simulink model "quadrotor_project_2021a"  (R2021a)
settings: Solver=VariableStepAuto  StartTime=0.0  StopTime=119.35  RelTol=1e-3
InitFcn:
  | sample_interval = 0.05;
  | Kp_z = 1000;
  | Kd_z = 10;
  | Kp_vel = 0.70;
  | Kd_vel = 0.2;
  | k1 = 65;
  | k2 = 25;
  | k3 = 65;
  | k4 = 25;
  | k5 = 60;
  | k6 = 55;
  | z_des = 5;
  | 
  | mdl_quadrotor;
  | J_x = quadrotor.J(1,1);
  | J_y = quadrotor.J(2,2);
  | J_z = quadrotor.J(3,3);
  | a1 = (J_y-J_z) / J_x;
  | a2 = (J_z-J_x) / J_y;
  | a3 = (J_x-J_y) / J_z;
  | b1 = 1 / J_x;
  | b2 = 1 / J_y;
  | b3 = 1 / J_z;
  | c1 = quadrotor.Ir / J_x;
  | c2 = quadrotor.Ir / J_y;
  | c3 = quadrotor.Ir / J_z;
undefined symbols (not defined in the file or in its folder): quadrotor, rot2, x_des, y_des
libraries: roblocks x4, simulink x1
settings Model: Creator=SPb19  LastModifiedBy=SPb19
settings SolverCC: ZeroCrossAlgorithm=Adaptive
settings DebuggingCC: UnconnectedInputMsg=none  UnconnectedOutputMsg=none  UnconnectedLineMsg=none
settings ModelReferenceCC: EnableRefExpFcnMdlSchedulingChecks=off
settings RTWCC: Description=Generic Real-Time Target  DLArmComputeVersion=20.02.1

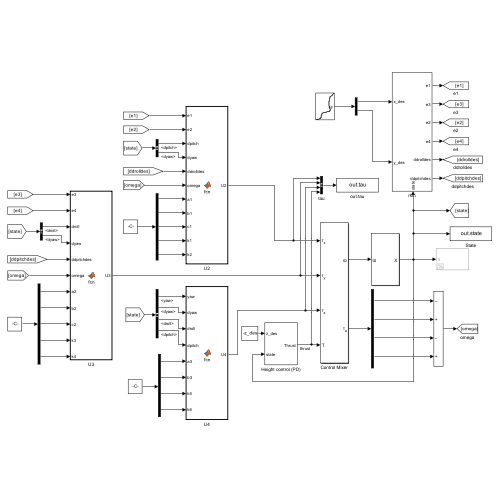
[thumbnail: Simulink's stored preview of the top-level diagram]
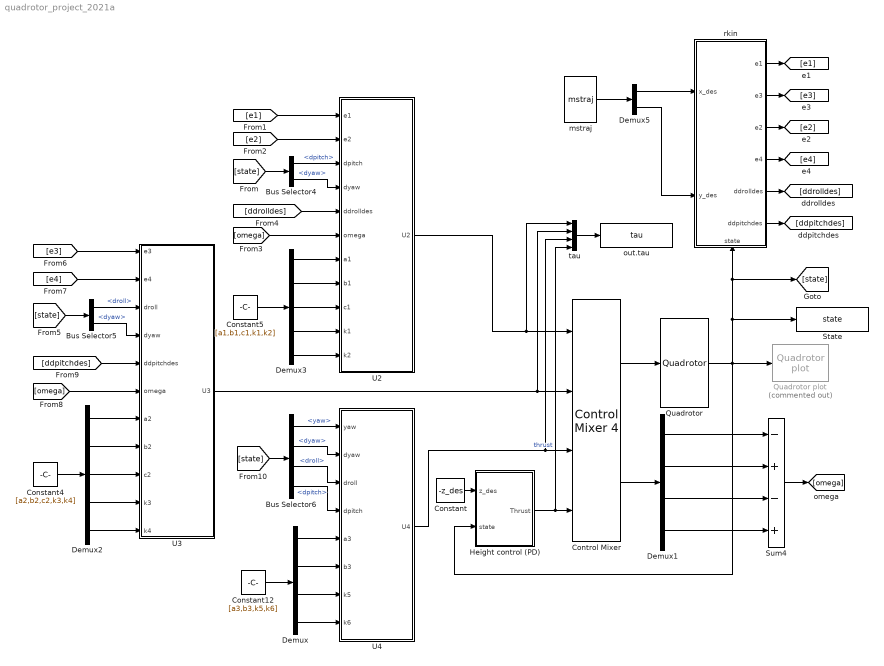
== system quadrotor_project_2021a ==
  Bus Selector4 : BusSelector  OutputSignals=dpitch,dyaw
  Bus Selector5 : BusSelector  OutputSignals=droll,dyaw
  Bus Selector6 : BusSelector  OutputSignals=yaw,dyaw,droll,dpitch
  Constant : Constant  Value=-z_des
  Constant12 : Constant  Value=[a3,b3,k5,k6]
  Constant4 : Constant  Value=[a2,b2,c2,k3,k4]
  Constant5 : Constant  Value=[a1,b1,c1,k1,k2]
  Control Mixer : roblocks/Vehicles/Control Mixer 4  quad=quadrotor  maxrot=1000  minrot=5
  Demux : Demux
  Demux1 : Demux
  Demux2 : Demux  Outputs=5
  Demux3 : Demux  Outputs=5
  Demux5 : Demux  Outputs=2
  Height control (PD) : Subsystem
  Quadrotor : roblocks/Vehicles/Quadrotor  quad=quadrotor  x0=[x_des(1), y_des(1) -z_des(1)]  groundflag=on
  Quadrotor plot : roblocks/Vehicles/Quadrotor plot  Commented=on  quad=quadrotor  xydim=100  zdim=10
  State : ToWorkspace  VariableName=state  SaveFormat=Timeseries  SampleTime=-1
  Sum4 : Sum  Inputs=-+-+
  U2 : MATLAB Function  TreatAsAtomicUnit=on
  U3 : MATLAB Function  TreatAsAtomicUnit=on
  U4 : MATLAB Function  TreatAsAtomicUnit=on
  mstraj : roblocks/Toolbox/mstraj  path=[x_des, y_des]  vaxis=[1 1]  tseg=[]  dt=sample_interval  tacc=0  setsimtime=on
  out.tau : ToWorkspace  VariableName=tau  SaveFormat=Timeseries  SampleTime=-1
  rkin : Subsystem
      settings: PortSchema="{\"entries\":[{\"content\":{\"sides\":[{\"content\":{\"connectorIds\":[\"In1\",\"In2\"]},\"type\":\"ConnectorPlacement.EquallySpacedRectSide\",\"uuid\":\"bc53fbe8-b9b1-4066-88ba-93360a1bcb5e\"},{\"content\":{\"connectorIds\":[\"Out1\",\"Out2\",\"Out3\",\"Out4\",\"Out5\",\"Out6\"],\"side\":\"RIGHT\"},\"type\":\"ConnectorPlacement.EquallySpacedRectSide\",\"uuid\":\"c29e6e71-3127-4518-8d0d-436f781ab69d\"},{\"content\":{\"connectorIds\":[],\"side\":\"TOP\"},\"type\":\"ConnectorPlacement.EquallySpacedRectSide\",\"uuid\":\"495c3253-bec1-47f4-9e26-6260d1e6c739\"},{\"content\":{\"connectorIds\":[\"In3\"],\"side\":\"BOTTOM\"},\"type\":\"ConnectorPlacement.EquallySpacedRectSide\",\"uuid\":\"80c5feda-b720-4a20-a958-e2d2e3b6db21\"}]},\"type\":\"ConnectorPlacement.EquallySpacedConnector\",\"uuid\":\"d02a51a0-9478-4fba-bb71-a1fe301afcd3\"}],\"packageUris\":[\"http://schema.mathworks.com/mf0/Connector/R2020b\"],\"version\":\"1.0\"}"
  tau : BusCreator  Inputs=4
  wires:
  Control Mixer/1 -> Quadrotor/1
  Height control (PD)/1(Thrust) -> tau/4, Control Mixer/4  "thrust"
  Quadrotor/1 -> Quadrotor plot/1, Height control (PD)/2(state), rkin/3(state), [state], State/1
  Constant/1 -> Height control (PD)/1(z_des)
  Control Mixer/2 -> Demux1/1
  Demux1/2 -> Sum4/2
  Demux1/3 -> Sum4/3
  Demux1/1 -> Sum4/1
  Demux1/4 -> Sum4/4
  Sum4/1 -> [omega]
  [state] -> Bus Selector4/1
  Bus Selector4/1 -> U2/3(dpitch)  "<dpitch>"
  Bus Selector4/2 -> U2/4(dyaw)  "<dyaw>"
  [e1] -> U2/1(e1)
  [e2] -> U2/2(e2)
  [omega] -> U2/6(omega)
  [ddrolldes] -> U2/5(ddrolldes)
  [e3] -> U3/1(e3)
  [state] -> Bus Selector5/1
  Bus Selector5/2 -> U3/4(dyaw)  "<dyaw>"
  [omega] -> U3/6(omega)
  [ddpitchdes] -> U3/5(ddpitchdes)
  Bus Selector5/1 -> U3/3(droll)  "<droll>"
  [e4] -> U3/2(e4)
  U3/1(U3) -> tau/2, Control Mixer/2
  [state] -> Bus Selector6/1
  Bus Selector6/1 -> U4/1(yaw)  "<yaw>"
  Bus Selector6/2 -> U4/2(dyaw)  "<dyaw>"
  Bus Selector6/3 -> U4/3(droll)  "<droll>"
  Bus Selector6/4 -> U4/4(dpitch)  "<dpitch>"
  rkin/1(e1) -> [e1]
  rkin/2(e3) -> [e3]
  rkin/3(e2) -> [e2]
  rkin/4(e4) -> [e4]
  rkin/5(ddrolldes) -> [ddrolldes]
  rkin/6(ddpitchdes) -> [ddpitchdes]
  Constant12/1 -> Demux/1
  Demux/1 -> U4/5(a3)
  Demux/2 -> U4/6(b3)
  Demux/3 -> U4/7(k5)
  Demux/4 -> U4/8(k6)
  Constant4/1 -> Demux2/1
  Demux2/1 -> U3/7(a2)
  Demux2/2 -> U3/8(b2)
  Demux2/3 -> U3/9(c2)
  Demux2/4 -> U3/10(k3)
  Demux2/5 -> U3/11(k4)
  Constant5/1 -> Demux3/1
  Demux3/1 -> U2/7(a1)
  Demux3/2 -> U2/8(b1)
  Demux3/3 -> U2/9(c1)
  Demux3/4 -> U2/10(k1)
  Demux3/5 -> U2/11(k2)
  Demux5/1 -> rkin/1(x_des)
  Demux5/2 -> rkin/2(y_des)
  U4/1(U4) -> tau/3, Control Mixer/3
  U2/1(U2) -> tau/1, Control Mixer/1
  mstraj/1 -> Demux5/1
  tau/1 -> out.tau/1

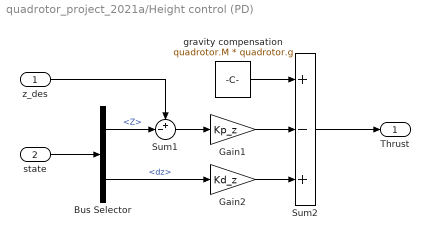
== system quadrotor_project_2021a/Height control (PD) ==
  z_des : Inport
  state : Inport  Port=2
  Bus Selector : BusSelector  OutputSignals=Z,dz
  Gain1 : Gain  Gain=Kp_z
  Gain2 : Gain  Gain=Kd_z
  Sum1 : Sum  Inputs=+-|
  Sum2 : Sum  Inputs=+-+
  gravity compensation : Constant  Value=quadrotor.M * quadrotor.g  SampleTime=0
  Thrust : Outport
  wires:
  Gain2/1 -> Sum2/3
  state/1 -> Bus Selector/1
  Bus Selector/1 -> Sum1/2  "<Z>"
  Gain1/1 -> Sum2/2
  Bus Selector/2 -> Gain2/1  "<dz>"
  z_des/1 -> Sum1/1
  gravity compensation/1 -> Sum2/1
  Sum1/1 -> Gain1/1
  Sum2/1 -> Thrust/1

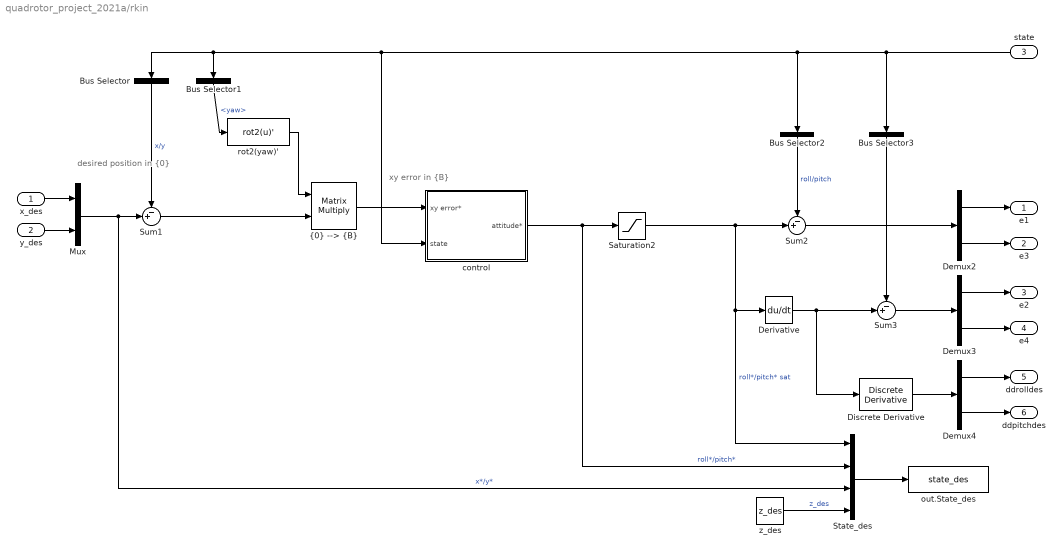
== system quadrotor_project_2021a/rkin ==
  note: xy error
      | in {B}
  note: desired position
      | in {0}
  x_des : Inport
  y_des : Inport  Port=2
  state : Inport  Port=3
  " control" : Subsystem  mask{P=Kp_vel, D=Kd_vel}
      mask prompts: P "Proportional gain"; D "Derivative gain"
  Bus Selector : BusSelector  OutputSignals=X,Y  OutputAsBus=on
  Bus Selector1 : BusSelector  OutputSignals=yaw
  Bus Selector2 : BusSelector  OutputSignals=roll,pitch  OutputAsBus=on
  Bus Selector3 : BusSelector  OutputSignals=droll,dpitch  OutputAsBus=on
  Demux2 : Demux  Outputs=2
  Demux3 : Demux  Outputs=2
  Demux4 : Demux  Outputs=2
  Derivative : Derivative
  Discrete Derivative : simulink/Discrete/Discrete Derivative  gainval=100  ICPrevScaledInput=0.0  OutMin=[]  OutMax=[]  OutDataType=fixdt(1, 16)  OutScaling=2^-10  DoSatur=off
  Mux : Mux  Inputs=2
  Saturation2 : Saturate  UpperLimit=deg2rad(25)  LowerLimit=deg2rad(-25)
  State_des : BusCreator  Inputs=4
  Sum1 : Sum  Inputs=-+|
  Sum2 : Sum  Inputs=-+|
  Sum3 : Sum  Inputs=-+|
  out.State_des : ToWorkspace  VariableName=state_des  SaveFormat=Timeseries  SampleTime=-1
  rot2(yaw)' : MATLABFcn  MATLABFcn=rot2(u)'  OutputDimensions=[2 2]  Output1D=off
  z_des : Constant  Value=z_des
  "{0} --> {B}" : Product  Multiplication=Matrix(*)  RndMeth=Zero
  e1 : Outport
  e3 : Outport  Port=2
  e2 : Outport  Port=3
  e4 : Outport  Port=4
  ddrolldes : Outport  Port=5
  ddpitchdes : Outport  Port=6
  wires:
  Sum3/1 -> Demux3/1
  Bus Selector/1 -> Sum1/1  "x/y"
  "{0} --> {B}"/1 -> " control"/1(xy error*)
  Demux3/2 -> e4/1
  Mux/1 -> State_des/3, Sum1/2  "x*/y*"
  state/1 -> Bus Selector3/1, Bus Selector1/1, Bus Selector/1, " control"/2(state), Bus Selector2/1
  rot2(yaw)'/1 -> "{0} --> {B}"/1
  Bus Selector2/1 -> Sum2/1  "roll/pitch"
  Derivative/1 -> Discrete Derivative/1, Sum3/2
  " control"/1(attitude*) -> State_des/2, Saturation2/1  "roll*/pitch*"
  Bus Selector3/1 -> Sum3/1
  Bus Selector1/1 -> rot2(yaw)'/1  "<yaw>"
  Demux2/1 -> e1/1
  y_des/1 -> Mux/2
  Sum1/1 -> "{0} --> {B}"/2
  Sum2/1 -> Demux2/1
  Demux4/1 -> ddrolldes/1
  Demux4/2 -> ddpitchdes/1
  Demux3/1 -> e2/1
  Demux2/2 -> e3/1
  x_des/1 -> Mux/1
  Discrete Derivative/1 -> Demux4/1
  Saturation2/1 -> Derivative/1, State_des/1, Sum2/2  "roll*/pitch* sat"
  State_des/1 -> out.State_des/1
  z_des/1 -> State_des/4  "z_des"

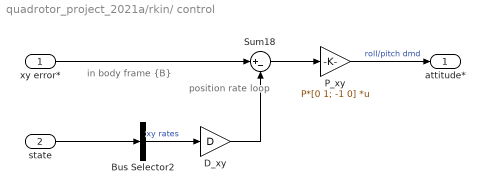
== system quadrotor_project_2021a/rkin/ control ==
  note: in body frame {B}
  note: position rate
      | loop
  xy error* : Inport
  state : Inport  Port=2
  Bus Selector2 : BusSelector  OutputSignals=dx,dy  OutputAsBus=on
  D_xy : Gain  Gain=D
  P_xy : Gain  Gain=P*[0 1; -1 0]  Multiplication=Matrix(K*u)
  Sum18 : Sum  Inputs=|+-
  attitude* : Outport
  wires:
  Bus Selector2/1 -> D_xy/1  "xy rates"
  D_xy/1 -> Sum18/2
  Sum18/1 -> P_xy/1
  xy error*/1 -> Sum18/1
  state/1 -> Bus Selector2/1
  P_xy/1 -> attitude*/1  "roll/pitch dmd"

== matlab function quadrotor_project_2021a/U3 ==
  data: e3 input; U3 output; e4 input; droll input; dyaw input; ddpitchdes input; omega input; a2 input; b2 input; c2 input; k3 input; k4 input
function U3 = fcn(e3,e4,droll,dyaw,ddpitchdes,omega,a2,b2,c2,k3,k4)

U3 = 1 / b2 * (e3 -...
                droll * dyaw * a2 -...
                c2 * droll * omega +...
                ddpitchdes -...
                k3 * (e4 + k3 * e3) -...
                k4 * e4);
end

== matlab function quadrotor_project_2021a/U2 ==
  data: e1 input; U2 output; e2 input; dpitch input; dyaw input; ddrolldes input; omega input; a1 input; b1 input; c1 input; k1 input; k2 input
function U2 = fcn(e1,e2,dpitch,dyaw,ddrolldes,omega,a1,b1,c1,k1,k2)

U2 = 1 / b1 * (e1 -...
                dpitch * dyaw * a1 +...
                c1 * dpitch * omega +...
                ddrolldes -...
                k1 * (e2 + k1 * e1) -...
                k2 * e2);
end

== matlab function quadrotor_project_2021a/U4 ==
  data: yaw input; dyaw input; droll input; U4 output; dpitch input; a3 input; b3 input; k5 input; k6 input
function U4 = fcn(yaw,dyaw,droll,dpitch,a3,b3,k5,k6)
ddyawdes = 0; 
dyaw_d = 0; 
yaw_d = 0;
e5 = yaw_d - yaw;
e6 = dyaw_d - dyaw;

U4 = 1 / b3 * (e5 -...
                droll * dpitch * a3 +...
                ddyawdes -...
                k5 * (e6 + k5 * e5) -...
                k6 * e6);
end
